simulink model "mcce"  (R2016a)
settings: Solver=VariableStepAuto  StartTime=0.0  StopTime=10.0  RelTol=1e-3
undefined symbols (not defined in the file): K, K_e, K_i
settings Model: Creator=manuel  LastModifiedBy=manuel

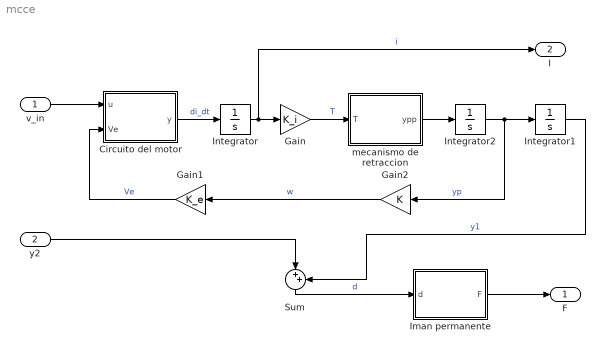
== system mcce ==
  v_in : Inport
  y2 : Inport  Port=2
  Circuito del motor : MATLAB Function  TreatAsAtomicUnit=on
  Gain : Gain  Gain=K_i
  Gain1 : Gain  Gain=K_e
  Gain2 : Gain  Gain=K
  Iman permanente : MATLAB Function  TreatAsAtomicUnit=on
  Integrator : Integrator
  Integrator1 : Integrator
  Integrator2 : Integrator
  Sum : Sum  Inputs=|++
  mecanismo de retraccion : MATLAB Function  TreatAsAtomicUnit=on
  F : Outport
  I : Outport  Port=2
  wires:
  v_in/1 -> Circuito del motor/1(u)
  Circuito del motor/1(y) -> Integrator/1  "di_dt"
  Integrator/1 -> I/1, Gain/1  "i"
  Gain/1 -> mecanismo de retraccion/1(T)  "T"
  Integrator2/1 -> Integrator1/1, Gain2/1  "yp"
  mecanismo de retraccion/1(ypp) -> Integrator2/1
  Gain1/1 -> Circuito del motor/2(Ve)  "Ve"
  Gain2/1 -> Gain1/1  "w"
  Sum/1 -> Iman permanente/1(d)  "d"
  Iman permanente/1(F) -> F/1
  y2/1 -> Sum/1
  Integrator1/1 -> Sum/2  "y1"

== matlab function mcce/mecanismo de retraccion ==
  data: T input; ypp output
function ypp = fcn(T)
%#codegen

ypp=T;

== matlab function mcce/Circuito del motor ==
  data: u input; y output; Ve input
function y = fcn(u,Ve)
%#codegen

y = u;

== matlab function mcce/Iman permanente ==
  data: d input; F output
function F = fcn(d)
%#codegen

F = d;
